simulink model "c28x_spi_interrupt_test_ert"  (R2021b)
settings: Solver=FixedStepDiscrete  StartTime=0.0  StopTime=inf  FixedStep=0.001  RelTol=1e-3  EnableMultiTasking=on
libraries: simulink x2, c280xlib x2, c2000lib x1, demo_controls x1
settings Model: SimulationMode=external  ExtModeTrigDuration=8  Creator=The MathWorks, Inc.  LastModifiedBy=The MathWorks, Inc.
settings SolverCC: AlgebraicLoopSolver=TrustRegion
settings DataIOCC: LimitDataPoints=on  SaveFormat=Array  SaveOutput=off  SaveTime=off  ReturnWorkspaceOutputs=off  SignalLoggingName=sigsOut
settings OptimizationCC: DefaultUnderspecifiedDataType=single  ExpressionDepthLimit=2147483647  InitFltsAndDblsToZero=on  LifeSpan=inf  MaxStackSize=512  EfficientTunableParamExpr=on
settings DebuggingCC: UnderspecifiedInitializationDetection=Classic  MergeDetectMultiDrivingBlocksExec=none  CheckExecutionContextPreStartOutputMsg=on  SignalResolutionControl=TryResolveAllWithWarning  MultiTaskDSMMsg=warning  MultiTaskCondExecSysMsg=none  SigSpecEnsureSampleTimeMsg=none  FcnCallInpInsideContextMsg=warning  AllowSymbolicDim=off  StateNameClashWarn=warning  SFUnexpectedBacktrackingDiag=warning  SFNoUnconditionalDefaultTransitionDiag=warning  SFExecutionAtInitializationDiag=none  SFMachineParentedDataDiag=warning  ArithmeticOperatorsInVariantConditions=warning
settings HardwareCC: ProdBitPerChar=16  ProdBitPerInt=16  ProdBitPerPointer=32  ProdBitPerSizeT=32  ProdBitPerPtrDiffT=32  ProdLargestAtomicInteger=Integer  ProdLargestAtomicFloat=None  ProdWordSize=16  ProdLongLongMode=on  ProdHWDeviceType=Texas Instruments->C2000  TargetBitPerChar=16  TargetBitPerInt=16  TargetBitPerPointer=16  TargetLargestAtomicInteger=Integer  TargetIntDivRoundTo=Zero  TargetEndianess=LittleEndian  TargetWordSize=16  TargetHWDeviceType=Texas Instruments->C2000  ProdEqTarget=off
settings ModelReferenceCC: UpdateModelReferenceTargets=IfOutOfDate  PropagateSignalLabelsOutOfModel=off
settings SFSimCC: SimUseLocalCustomCode=off  CustomCodeUndefinedFunction=UseInterfaceOnly
settings RTWCC: Description=Embedded Coder  SystemTargetFile=ert.tlc  HardwareBoard=TI Delfino F28379D LaunchPad  TemplateMakefile=ert_default_tmf  PostCodeGenCommand=; codertarget.postCodeGenHookCommand(h)  RTWUseLocalCustomCode=off  Toolchain=Texas Instruments Code Composer Studio (C2000)
settings CodeAppCC: IgnoreCustomStorageClasses=off  CustomSymbolStrType=$N$R$M  StateflowObjectComments=on  InternalIdentifier=Classic
settings ERTTargetCC: CodeReplacementLibrary=TI C28x  MultiwordLength=2048  ParMdlRefBuildCompliant=off  CompOptLevelCompliant=off  ConcurrentExecutionCompliant=off  CPPClassGenCompliant=off  ExtModeTransport=4  ExtModeStaticAlloc=on  ExtModeStaticAllocSize=2048  ExtModeMexFile=ext_xcp  ExtModeIntrfLevel=Level2 - Open  ConvertIfToSwitch=off  SuppressUnreachableDefaultCases=off
settings ConfigComp: CovMetricSettings=dw  CovSaveCumulativeToWorkspaceVar=on  CovSaveSingleToWorkspaceVar=on  CovExternalEMLEnable=off  CovSFcnEnable=off

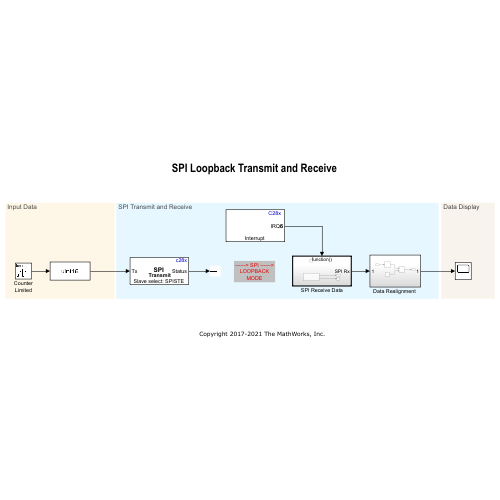
[thumbnail: Simulink's stored preview of the top-level diagram]
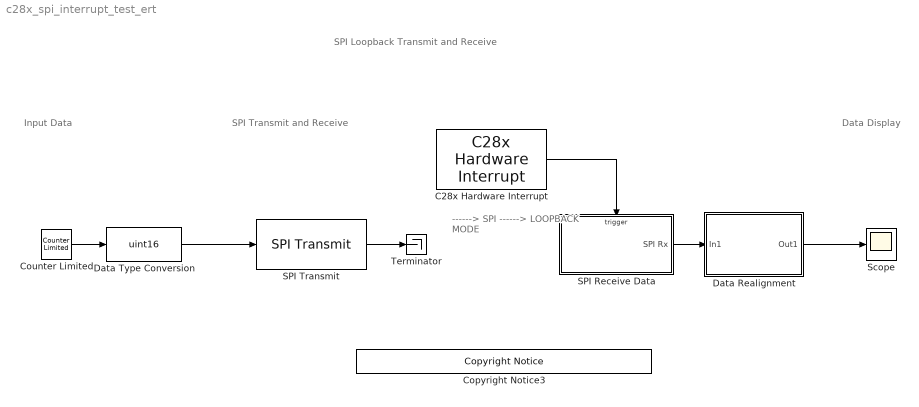
== system c28x_spi_interrupt_test_ert ==
  note: SPI Loopback Transmit and Receive
  note: Input Data
  note: SPI Transmit and Receive
  note: ------> SPI ------>
      | LOOPBACK
      | MODE
  note: Data Display
  C28x Hardware Interrupt : c2000lib/Scheduling/C28x Hardware Interrupt  irqnumbers=6  pienumbers=1  irqpriorities=30  irqpreempts=1  showinput=off  dspchiptype=C280X
      settings: SourceProductBaseCode=TIC2000
  Copyright Notice3 : demo_controls/Copyright Notice  year=2017  prod=tic2000
      settings: SourceProductBaseCode=ME
  Counter Limited : simulink/Sources/Counter Limited  uplimit=255  tsamp=0.1
  "Data Realignment " : Subsystem
  Data Type Conversion : DataTypeConversion  OutDataTypeStr=uint16
  SPI Receive Data : Subsystem
  SPI Transmit : c280xlib/SPI Transmit  SPISelect=SPI_A  ClockPolarity=Rising_edge  ClockPhase=No_delay  SPIModule=uint32(0)  Mode=Master  BusSpeed=uint32(1000000)  FirstBitToTransfer=Most significant bit (MSB)  ClockMode=0  BlockFunction=Write  EnableRegisterAddress=on  RegisterAddress=0  OutputDataType=int8  OutputDataLength=1  BlockingMode=off  DataBits=16  UseCustomSSPin=Provided by the SPI peripheral  ActiveLowSSPin=Active low  Pin=0
      settings: SourceProductBaseCode=TIC2000
  Scope : Scope
  Terminator : Terminator
  wires:
  Counter Limited/1 -> Data Type Conversion/1
  SPI Transmit/1 -> Terminator/1
  Data Type Conversion/1 -> SPI Transmit/1
  C28x Hardware Interrupt/1 -> SPI Receive Data/Trigger
  SPI Receive Data/1(SPI Rx) -> "Data Realignment "/1(In1)
  "Data Realignment "/1(Out1) -> Scope/1

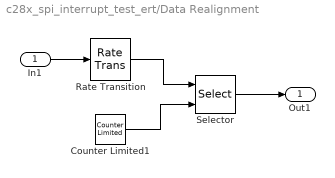
== system c28x_spi_interrupt_test_ert/Data Realignment  ==
  In1 : Inport
  Counter Limited1 : simulink/Sources/Counter Limited  uplimit=3  tsamp=0.1
  Rate Transition : RateTransition  Deterministic=off  OutPortSampleTime=0.1
  Selector : Selector  IndexMode=Zero-based  InputPortWidth=4  IndexOptions=Index vector (port)  Indices=1  OutputSizes=1
  Out1 : Outport  VectorParamsAs1DForOutWhenUnconnected=off
  wires:
  Rate Transition/1 -> Selector/1
  In1/1 -> Rate Transition/1
  Selector/1 -> Out1/1
  Counter Limited1/1 -> Selector/2

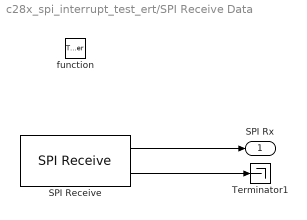
== system c28x_spi_interrupt_test_ert/SPI Receive Data ==
  function : TriggerPort  TriggerType=function-call  VariantControl=Variant
  SPI Receive : c280xlib/SPI Receive  SPISelect=SPI_A  ClockPolarity=Rising_edge  ClockPhase=No_delay  SPIModule=uint32(0)  Mode=Master  BusSpeed=uint32(1000000)  FirstBitToTransfer=Most significant bit (MSB)  ClockMode=0  BlockFunction=Read  EnableRegisterAddress=on  RegisterAddress=0  OutputDataType=uint16  OutputDataLength=4  BlockingMode=off  SampleTime=-1  DataBits=16  UseCustomSSPin=Provided by the SPI peripheral  ActiveLowSSPin=Active low  Pin=0
      settings: SourceProductBaseCode=TIC2000
  Terminator1 : Terminator
  SPI Rx : Outport  VectorParamsAs1DForOutWhenUnconnected=off
  wires:
  SPI Receive/2 -> Terminator1/1
  SPI Receive/1 -> SPI Rx/1
